simulink model "MHH_BUOI2_bai2"  (R2020b)
settings: Solver=VariableStepAuto  StartTime=0.0  StopTime=10  MaxStep=0.01  RelTol=1e-3
values from neighbouring files (symbols this model uses):
  b = 0.2    [bai4.mat]
  k = 10    [bai4.mat]
  M = 1    [bai4.mat]
settings Model: Creator=John Andrew  LastModifiedBy=John Andrew

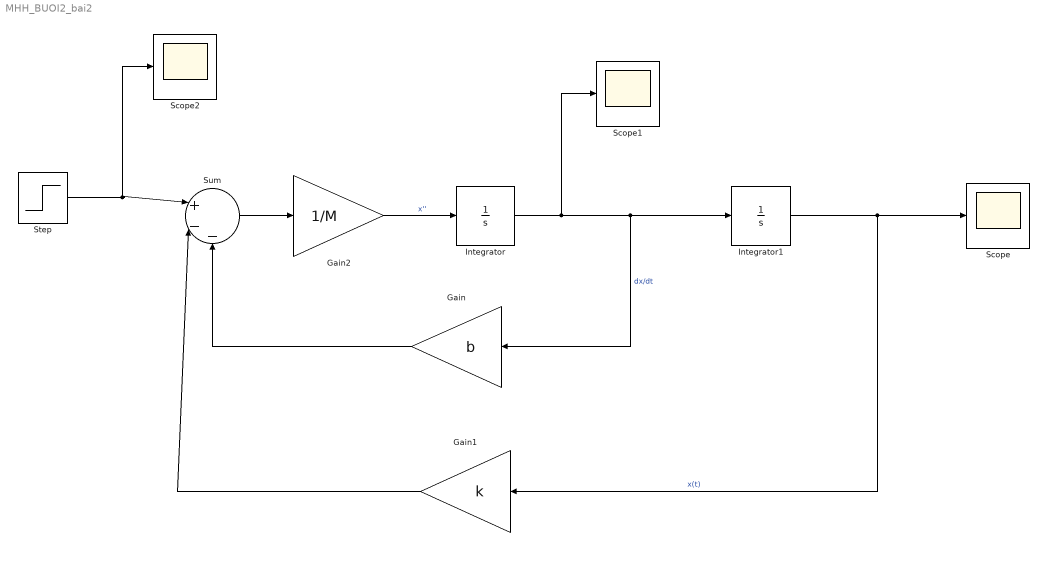
== system MHH_BUOI2_bai2 ==
  Gain : Gain  Gain=b
  Gain1 : Gain  Gain=k
  Gain2 : Gain  Gain=1/M
  Integrator : Integrator
  Integrator1 : Integrator
  Scope : Scope
  Scope1 : Scope
  Scope2 : Scope
  Step : Step  SampleTime=0
  Sum : Sum  Inputs=|+--
  wires:
  Gain/1 -> Sum/3
  Step/1 -> Scope2/1, Sum/1
  Gain1/1 -> Sum/2
  Sum/1 -> Gain2/1
  Gain2/1 -> Integrator/1  "x''"
  Integrator/1 -> Scope1/1, Gain/1, Integrator1/1  "dx/dt"
  Integrator1/1 -> Gain1/1, Scope/1  "x(t)"
